simulink model "Centro_contra_desplazado"  (R2016a)
settings: Solver=VariableStepAuto  StartTime=0.0  StopTime=10.0  RelTol=1e-3
undefined symbols (not defined in the file or in its folder): sigbuilder_block
settings Model: Creator=daniel  LastModifiedBy=daniel
settings DataIOCC: LimitDataPoints=on
settings DebuggingCC: AllowSymbolicDim=off
settings ModelReferenceCC: PropagateSignalLabelsOutOfModel=off
settings GRTTargetCC: GeneratePreprocessorConditionals=Use local settings

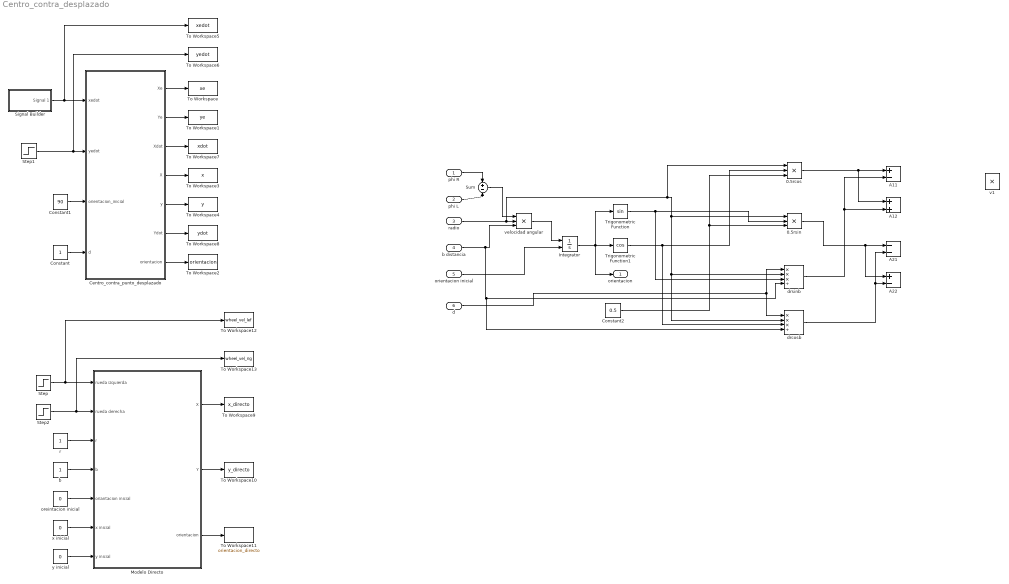
== system Centro_contra_desplazado ==
  phi R : Inport
  phi L : Inport  Port=2
  radio : Inport  Port=3
  b distancia : Inport  Port=4
  orientacion inicial : Inport  Port=5
  d : Inport  Port=6
  0.5rcos : Product  Inputs=3
  0.5rsin : Product  Inputs=3
  A11 : Sum  Inputs=+-
  A12 : Sum
  A21 : Sum  Inputs=--
  A22 : Sum  Inputs=+-
  Centro_contra_punto_desplazado : Subsystem
  Constant : Constant
  Constant1 : Constant  Value=90
  Constant2 : Constant  Value=0.5
  Integrator : Integrator  InitialConditionSource=external
  Modelo Directo : Subsystem
  Signal Builder : Subsystem  Tag=STV Subsys  LoadFcn=sigbuilder_block('load');  StartFcn=sigbuilder_block('start');  StopFcn=sigbuilder_block('stop');  ClipboardFcn=sigbuilder_block('clipboard');  mask(Sigbuilder block){}
      mask help: Simulink:masks:SigbuilderBlock_MD
      mask init:
      | if ~strcmp(get_param(bdroot(gcbh),'SimulationStatus'),'stopped') tuvar = sigbuilder_block('maskInit'); end
      settings: CopyFcn=sigbuilder_block('copy');  DeleteFcn=sigbuilder_block('delete');  ModelCloseFcn=sigbuilder_block('modelClose');  PreSaveFcn=sigbuilder_block('preSave');  PauseFcn=sigbuilder_block('pause');  ContinueFcn=sigbuilder_block('continue');  NameChangeFcn=sigbuilder_block('namechange');  OpenFcn=sigbuilder_block('open',[197.25 99.75 550.5 358.5 ]);  CloseFcn=sigbuilder_block('close');
      mask Display: plot(0, 0, 100, 100,[2, 2, 32, 32, 2], [68, 8, 8, 68, 68],[32, 2], [38, 38], [32, 19, 2],[53, 60, 44], [32, 17, 17, 2],[16, 16, 31, 31]);txt = getActiveGroup(gcbh);text(2, 100, txt,'verticalAlignment', 'top');
  Step : Step  SampleTime=0
  Step1 : Step  SampleTime=0
  Step2 : Step  Time=5  SampleTime=0
  Sum : Sum  Inputs=+-
  To Workspace : ToWorkspace  VariableName=xe  SaveFormat=Timeseries  SampleTime=-1
  To Workspace1 : ToWorkspace  VariableName=ye  SaveFormat=Timeseries  SampleTime=-1
  To Workspace10 : ToWorkspace  VariableName=y_directo  SaveFormat=Timeseries  SampleTime=-1
  To Workspace11 : ToWorkspace  VariableName=orientacion_directo  SaveFormat=Timeseries  SampleTime=-1
  To Workspace12 : ToWorkspace  VariableName=wheel_vel_lef  SaveFormat=Timeseries  SampleTime=-1
  To Workspace13 : ToWorkspace  VariableName=wheel_vel_rig  SaveFormat=Timeseries  SampleTime=-1
  To Workspace2 : ToWorkspace  VariableName=orientacion  SaveFormat=Timeseries  SampleTime=-1
  To Workspace3 : ToWorkspace  VariableName=x  SaveFormat=Timeseries  SampleTime=-1
  To Workspace4 : ToWorkspace  VariableName=y  SaveFormat=Timeseries  SampleTime=-1
  To Workspace5 : ToWorkspace  VariableName=xedot  SaveFormat=Timeseries  SampleTime=-1
  To Workspace6 : ToWorkspace  VariableName=yedot  SaveFormat=Timeseries  SampleTime=-1
  To Workspace7 : ToWorkspace  VariableName=xdot  SaveFormat=Timeseries  SampleTime=-1
  To Workspace8 : ToWorkspace  VariableName=ydot  SaveFormat=Timeseries  SampleTime=-1
  To Workspace9 : ToWorkspace  VariableName=x_directo  SaveFormat=Timeseries  SampleTime=-1
  Trigonometric Function : Trigonometry
  Trigonometric Function1 : Trigonometry  Operator=cos
  b : Constant
  drcosb : Product  Inputs=***/
  drsinb : Product  Inputs=***/
  oreintacion inicial : Constant  Value=0
  r : Constant
  v1 : Product
  velocidad angular : Product  Inputs=3
  x inicial : Constant  Value=0
  y inicial : Constant  Value=0
  orientacion : Outport
  wires:
  Signal Builder/1(Signal 1) -> To Workspace5/1, Centro_contra_punto_desplazado/1(xedot)
  Step1/1 -> Centro_contra_punto_desplazado/2(yedot), To Workspace6/1
  Constant1/1 -> Centro_contra_punto_desplazado/3(orientacion_inicial)
  Constant/1 -> Centro_contra_punto_desplazado/4(d)
  Centro_contra_punto_desplazado/1(Xe) -> To Workspace/1
  Centro_contra_punto_desplazado/2(Ye) -> To Workspace1/1
  Centro_contra_punto_desplazado/3(Xdot) -> To Workspace7/1
  Centro_contra_punto_desplazado/4(X) -> To Workspace3/1
  Centro_contra_punto_desplazado/5(y) -> To Workspace4/1
  Centro_contra_punto_desplazado/6(Ydot) -> To Workspace8/1
  Centro_contra_punto_desplazado/7(orientacion) -> To Workspace2/1
  Step2/1 -> To Workspace13/1, Modelo Directo/2(rueda derecha)
  Step/1 -> Modelo Directo/1(rueda izquierda), To Workspace12/1
  r/1 -> Modelo Directo/3(r)
  b/1 -> Modelo Directo/4(b)
  oreintacion inicial/1 -> Modelo Directo/5(oriantacion inicial)
  x inicial/1 -> Modelo Directo/6(x inicial)
  y inicial/1 -> Modelo Directo/7(y inicial)
  Modelo Directo/1(X) -> To Workspace9/1
  Modelo Directo/2(Y) -> To Workspace10/1
  Modelo Directo/3(orientacion) -> To Workspace11/1
  phi R/1 -> Sum/1
  phi L/1 -> Sum/2
  radio/1 -> drcosb/2, drsinb/2, 0.5rsin/1, 0.5rcos/1, velocidad angular/2
  b distancia/1 -> drcosb/4, drsinb/4, velocidad angular/3
  Sum/1 -> velocidad angular/1
  velocidad angular/1 -> Integrator/1
  orientacion inicial/1 -> Integrator/2
  Integrator/1 -> Trigonometric Function/1, Trigonometric Function1/1, orientacion/1
  Constant2/1 -> 0.5rcos/3, 0.5rsin/3
  Trigonometric Function/1 -> drsinb/3, 0.5rsin/2
  Trigonometric Function1/1 -> drcosb/3, 0.5rcos/2
  d/1 -> drsinb/1, drcosb/1
  0.5rcos/1 -> A12/1, A11/1
  drsinb/1 -> A12/2, A11/2
  0.5rsin/1 -> A22/1, A21/1
  drcosb/1 -> A22/2, A21/2

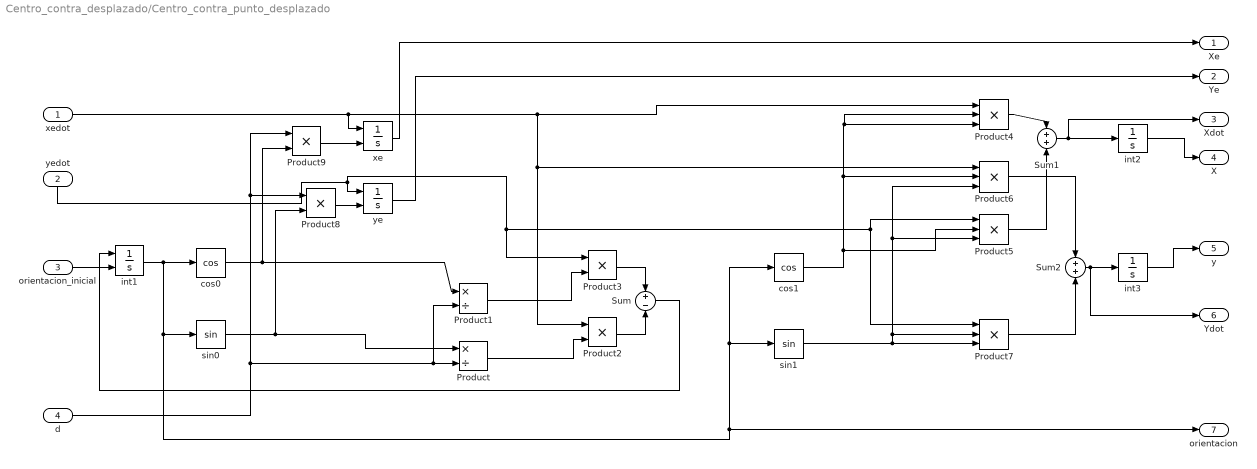
== system Centro_contra_desplazado/Centro_contra_punto_desplazado ==
  xedot : Inport
  yedot : Inport  Port=2
  orientacion_inicial : Inport  Port=3
  d : Inport  Port=4
  Product : Product  Inputs=*/
  Product1 : Product  Inputs=*/
  Product{2..3,8..9} (4 alike) : Product
  Product{4..7} (4 alike) : Product  Inputs=3
  Sum : Sum  Inputs=+-
  Sum1 : Sum
  Sum2 : Sum
  cos0 : Trigonometry  Operator=cos
  "cos1 " : Trigonometry  Operator=cos
  int1 : Integrator  InitialConditionSource=external
  int2 : Integrator
  int3 : Integrator
  sin0 : Trigonometry
  "sin1 " : Trigonometry
  xe : Integrator  InitialConditionSource=external  InitialCondition=1
  ye : Integrator  InitialConditionSource=external
  Xe : Outport
  Ye : Outport  Port=2
  Xdot : Outport  Port=3
  X : Outport  Port=4
  y : Outport  Port=5
  Ydot : Outport  Port=6
  orientacion : Outport  Port=7
  wires:
  Product2/1 -> Sum/2
  xedot/1 -> xe/1, Product4/1, Product6/1, Product2/1
  Product4/1 -> Sum1/1
  xe/1 -> Xe/1
  int3/1 -> y/1
  Product7/1 -> Sum2/2
  Sum2/1 -> Ydot/1, int3/1
  int1/1 -> cos0/1, sin0/1, orientacion/1, "sin1 "/1, "cos1 "/1
  Sum1/1 -> Xdot/1, int2/1
  yedot/1 -> Product5/1, Product7/1, Product3/1, ye/1
  orientacion_inicial/1 -> int1/2
  d/1 -> Product8/1, Product9/1, Product1/2, Product/2
  Product8/1 -> ye/2
  cos0/1 -> Product9/2, Product1/1
  "sin1 "/1 -> Product5/3, Product6/3, Product7/2, Product7/3
  Product9/1 -> xe/2
  Sum/1 -> int1/1
  Product6/1 -> Sum2/1
  Product1/1 -> Product3/2
  Product3/1 -> Sum/1
  int2/1 -> X/1
  "cos1 "/1 -> Product6/2, Product4/2, Product4/3, Product5/2
  Product/1 -> Product2/2
  Product5/1 -> Sum1/2
  sin0/1 -> Product8/2, Product/1
  ye/1 -> Ye/1

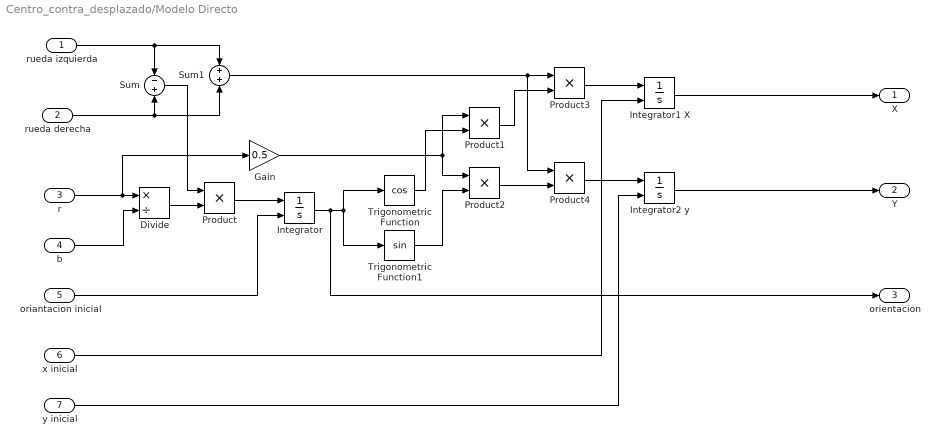
== system Centro_contra_desplazado/Modelo Directo ==
  rueda izquierda : Inport
  rueda derecha : Inport  Port=2
  r : Inport  Port=3
  b : Inport  Port=4
  oriantacion inicial : Inport  Port=5
  x inicial : Inport  Port=6
  y inicial : Inport  Port=7
  Divide : Product  Inputs=*/
  Gain : Gain  Gain=0.5
  Integrator : Integrator  InitialConditionSource=external
  Integrator1 X : Integrator  InitialConditionSource=external
  Integrator2 y : Integrator  InitialConditionSource=external
  Product{,1..4} (5 alike) : Product
  Sum : Sum  Inputs=-+
  Sum1 : Sum
  Trigonometric Function : Trigonometry  Operator=cos  OutputSignalType=real
  Trigonometric Function1 : Trigonometry  OutputSignalType=real
  X : Outport
  Y : Outport  Port=2
  orientacion : Outport  Port=3
  wires:
  r/1 -> Gain/1, Divide/1
  oriantacion inicial/1 -> Integrator/2
  Sum1/1 -> Product3/1, Product4/1
  Integrator/1 -> orientacion/1, Trigonometric Function1/1, Trigonometric Function/1
  rueda derecha/1 -> Sum/2, Sum1/2
  Sum/1 -> Product/1
  b/1 -> Divide/2
  Integrator1 X/1 -> X/1
  Integrator2 y/1 -> Y/1
  Trigonometric Function1/1 -> Product2/2
  Gain/1 -> Product1/1, Product2/1
  x inicial/1 -> Integrator1 X/2
  Product4/1 -> Integrator2 y/1
  Product/1 -> Integrator/1
  Trigonometric Function/1 -> Product1/2
  Product2/1 -> Product4/2
  rueda izquierda/1 -> Sum1/1, Sum/1
  Product1/1 -> Product3/2
  Product3/1 -> Integrator1 X/1
  Divide/1 -> Product/2
  y inicial/1 -> Integrator2 y/2

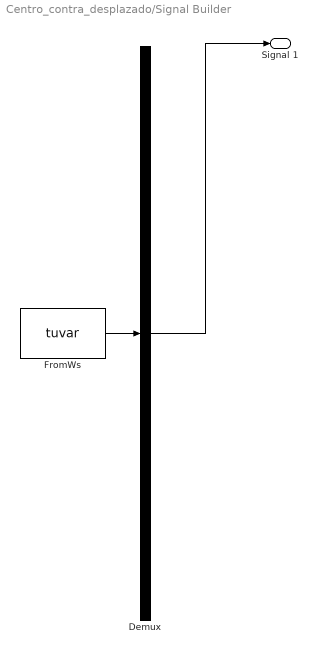
== system Centro_contra_desplazado/Signal Builder ==
  Demux : Demux  Tag=STV Demux  Outputs=1
  FromWs : FromWorkspace  Tag=STV FromWs  VariableName=tuvar  SampleTime=0
      SigBuilderData=|
      | common.afterFinalStr = 'Extrapolate'
      | common.sampleTime = 0
      | dataSet.timeRange = [0 10]
      | dataSet.name = 'Group 1'
      | sbobj.Groups.Name = 'Group 1'
      | sbobj.Groups.Signals.Name = 'Signal 1'
      | sbobj.Groups.Signals.XData = [0 2.3 2.3 4.28 4.28 10]
      | sbobj.Groups.Signals.YData = [0 0 1 1 0 0]
  Signal 1 : Outport  Tag=STV Outport
  wires:
  Demux/1 -> Signal 1/1
  FromWs/1 -> Demux/1
